simulink model "bipedal_robot"  (R2020b)
settings: Solver=ode23  StartTime=0.0  StopTime=TG.Tsim  MaxStep=0.01  RelTol=1e-3  AbsTol=1e-3  EnableMultiTasking=on
values from neighbouring files (symbols this model uses):
  cdf_data = zmp_cdf(foot,total_mass,0)    [bipedal.m]
  g = 9.80665    [bipedal.m]
  Tfil = Ts*10    (= 0.01)    [bipedal.m]
  total_mass = mlist(1) + ll_mass + rl_mass    [bipedal.m]
  Ts = 1/fs    (= 0.001)    [bipedal.m]
  use_reference_FBdata = 0    [bipedal.m]
undefined symbols (not defined in the file or in its folder): Base, ctrl_cfg_rem, ctrl_config, ctrl_data, foot, LefAnklePitch, LefAnkleRoll, LefHipPitch, LefHipRoll, LefHipYaw, LefKnee, lleg_FS_str, lleg_str, RigAnklePitch, RigAnkleRoll, RigHipPitch, RigHipRoll, RigHipYaw, RigKnee, rleg_FS_str, rleg_str, sim_floor, TG_test_type, X, Y, Z
libraries: sm_lib x49, biped_lib x36, nesl_utility x9, robotmaniplib x5, controller_lib x1, simulink x1, Contact_Forces_Lib x1
(part 3 of 3)

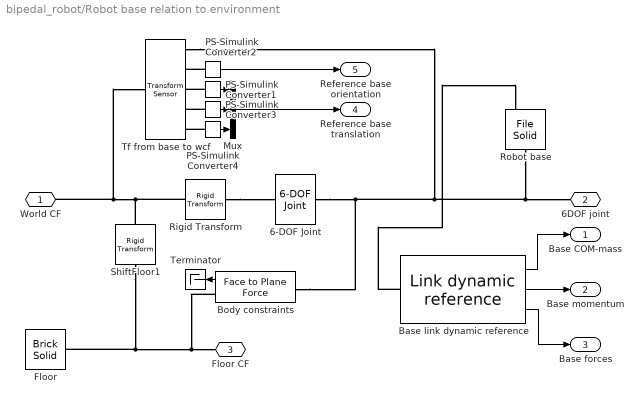
== system bipedal_robot/Robot base relation to environment ==
  6-DOF Joint : sm_lib/Joints/6-DOF Joint  JointMode=Normal  SenseConstraintForce=off  SenseConstraintForceX=off  SenseConstraintForceY=off  SenseConstraintForceZ=off  SenseConstraintTorque=off  SenseConstraintTorqueX=off  SenseConstraintTorqueY=off  SenseConstraintTorqueZ=off  SenseTotalForce=off  SenseTotalForceX=off  SenseTotalForceY=off  SenseTotalForceZ=off  SenseTotalTorque=off  SenseTotalTorqueX=off  SenseTotalTorqueY=off  SenseTotalTorqueZ=off  CompositeWrenchDir=FollowerOnBase  CompositeWrenchFrame=BaseFrame  PxEquilibriumPosition=0  PxEquilibriumPositionUnits=m  PxSpringStiffness=0  PxSpringStiffnessUnits=N/m  PxDampingCoefficient=0  PxDampingCoefficientUnits=N/(m/s)  PxTorqueActuationMode=NoTorque  PxMotionActuationMode=ComputedMotion  PxSensePosition=off  PxSenseVelocity=off  PxSenseAcceleration=off  PxSenseTorqueForce=off  PxSenseLowerLimitTorqueForce=off  PxSenseUpperLimitTorqueForce=off  PxLowerLimitSpecify=off  PxLowerLimitBound=-1  PxLowerLimitBoundUnits=m  PxLowerLimitStiffness=1e6  PxLowerLimitStiffnessUnits=N/m  PxLowerLimitDamping=1e3  PxLowerLimitDampingUnits=N/(m/s)  PxLowerLimitTransitionRegionWidth=1e-4  PxLowerLimitTransitionRegionWidthUnits=m  PxUpperLimitSpecify=off  PxUpperLimitBound=1  PxUpperLimitBoundUnits=m  PxUpperLimitStiffness=1e6  PxUpperLimitStiffnessUnits=N/m  PxUpperLimitDamping=1e3  PxUpperLimitDampingUnits=N/(m/s)  PxUpperLimitTransitionRegionWidth=1e-4  PxUpperLimitTransitionRegionWidthUnits=m  PxPositionTargetSpecify=on  PxPositionTargetPriority=High  PxPositionTargetValue=Base.Xinit(1)  PxPositionTargetValueUnits=m  PxVelocityTargetSpecify=off  PxVelocityTargetPriority=High  PxVelocityTargetValue=0  PxVelocityTargetValueUnits=m/s  PyEquilibriumPosition=0  PyEquilibriumPositionUnits=m  PySpringStiffness=0  PySpringStiffnessUnits=N/m  PyDampingCoefficient=0  PyDampingCoefficientUnits=N/(m/s)  PyTorqueActuationMode=NoTorque  PyMotionActuationMode=ComputedMotion  PySensePosition=off  PySenseVelocity=off  PySenseAcceleration=off  PySenseTorqueForce=off  PySenseLowerLimitTorqueForce=off  PySenseUpperLimitTorqueForce=off  PyLowerLimitSpecify=off  PyLowerLimitBound=-1  PyLowerLimitBoundUnits=m  PyLowerLimitStiffness=1e6  PyLowerLimitStiffnessUnits=N/m  PyLowerLimitDamping=1e3  PyLowerLimitDampingUnits=N/(m/s)  PyLowerLimitTransitionRegionWidth=1e-4  PyLowerLimitTransitionRegionWidthUnits=m  PyUpperLimitSpecify=off  PyUpperLimitBound=1  PyUpperLimitBoundUnits=m  PyUpperLimitStiffness=1e6  PyUpperLimitStiffnessUnits=N/m  PyUpperLimitDamping=1e3  PyUpperLimitDampingUnits=N/(m/s)  PyUpperLimitTransitionRegionWidth=1e-4  PyUpperLimitTransitionRegionWidthUnits=m  PyPositionTargetSpecify=on  PyPositionTargetPriority=High  PyPositionTargetValue=Base.Xinit(2)  PyPositionTargetValueUnits=m  PyVelocityTargetSpecify=off  PyVelocityTargetPriority=High  PyVelocityTargetValue=0  PyVelocityTargetValueUnits=m/s  PzEquilibriumPosition=0  PzEquilibriumPositionUnits=m  PzSpringStiffness=0  PzSpringStiffnessUnits=N/m  PzDampingCoefficient=0  PzDampingCoefficientUnits=N/(m/s)  PzTorqueActuationMode=NoTorque  PzMotionActuationMode=ComputedMotion  PzSensePosition=off  PzSenseVelocity=off  PzSenseAcceleration=off  PzSenseTorqueForce=off  PzSenseLowerLimitTorqueForce=off  PzSenseUpperLimitTorqueForce=off  PzLowerLimitSpecify=off  PzLowerLimitBound=0  PzLowerLimitBoundUnits=m  PzLowerLimitStiffness=1e6  PzLowerLimitStiffnessUnits=N/m  PzLowerLimitDamping=1e3  PzLowerLimitDampingUnits=N/(m/s)  PzLowerLimitTransitionRegionWidth=1e-4  PzLowerLimitTransitionRegionWidthUnits=m  PzUpperLimitSpecify=off  PzUpperLimitBound=1  PzUpperLimitBoundUnits=m  PzUpperLimitStiffness=1e6  PzUpperLimitStiffnessUnits=N/m  PzUpperLimitDamping=1e3  PzUpperLimitDampingUnits=N/(m/s)  PzUpperLimitTransitionRegionWidth=1e-4  PzUpperLimitTransitionRegionWidthUnits=m  PzPositionTargetSpecify=on  PzPositionTargetPriority=High  PzPositionTargetValue=Base.Xinit(3)  PzPositionTargetValueUnits=m  PzVelocityTargetSpecify=off  PzVelocityTargetPriority=High  PzVelocityTargetValue=0  PzVelocityTargetValueUnits=m/s  SphDefPosRotationMethod=None  SphDefPosRotationAngleUnits=deg  SphDefPosRotationStandardAxis=+Z  SphDefPosRotationAngle=0.0  SphDefPosRotationArbitraryAxis=[0 0 1]  SphDefPosFollAlignAxisA=+X  SphDefPosBaseAlignAxisA=+Y  SphDefPosFollAlignAxisB=+Y  SphDefPosBaseAlignAxisB=+Z  SphDefPosRotationSequenceAxes=FollowerAxes  SphDefPosRotationSequence=XYX  SphDefPosRotationSequenceAngles=[0 0 0]  SphDefPosRotationSequenceAnglesUnits=deg  SphDefPosRotationMatrix=[1 0 0; 0 1 0; 0 0 1]  SphEqPosRotationMethod=None  SphEqPosRotationAngleUnits=deg  SphEqPosRotationStandardAxis=+Z  SphEqPosRotationAngle=0.0  SphEqPosRotationArbitraryAxis=[0 0 1]  SphEqPosFollAlignAxisA=+X  SphEqPosBaseAlignAxisA=+Y  SphEqPosFollAlignAxisB=+Y  SphEqPosBaseAlignAxisB=+Z  SphEqPosRotationSequenceAxes=FollowerAxes  SphEqPosRotationSequence=XYX  SphEqPosRotationSequenceAngles=[0 0 0]  SphEqPosRotationSequenceAnglesUnits=deg  SphEqPosRotationMatrix=[1 0 0; 0 1 0; 0 0 1]  SphSpringStiffness=0  SphSpringStiffnessUnits=N*m/deg  SphDampingCoefficient=0  SphDampingCoefficientUnits=N*m/(deg/s)  SphActuateTorqueX=off  SphActuateTorqueY=off  SphActuateTorqueZ=off  SphActuateTorque=off  SphTorqueActuationMode=NoTorque  SphMotionActuationMode=ComputedMotion  SphActuationFrame=BaseFrame  SphSensePosition=off  SphSenseVelocityX=off  SphSenseVelocityY=off  SphSenseVelocityZ=off  SphSenseVelocity=off  SphSenseAccelerationX=off  SphSenseAccelerationY=off  SphSenseAccelerationZ=off  SphSenseAcceleration=off  SphSenseTorqueX=off  SphSenseTorqueY=off  SphSenseTorqueZ=off  SphSenseTorqueForce=off  SphSenseLowerLimitTorqueMag=off  SphSenseUpperLimitTorqueMag=off  SphSensingFrame=BaseFrame  SphLowerLimitSpecify=off  SphLowerLimitBound=15  SphLowerLimitBoundUnits=deg  SphLowerLimitStiffness=1e4  SphLowerLimitStiffnessUnits=N*m/deg  SphLowerLimitDamping=10  SphLowerLimitDampingUnits=N*m/(deg/s)  SphLowerLimitTransitionRegionWidth=0.1  SphLowerLimitTransitionRegionWidthUnits=deg  SphUpperLimitSpecify=off  SphUpperLimitBound=45  SphUpperLimitBoundUnits=deg  SphUpperLimitStiffness=1e4  SphUpperLimitStiffnessUnits=N*m/deg  SphUpperLimitDamping=10  SphUpperLimitDampingUnits=N*m/(deg/s)  SphUpperLimitTransitionRegionWidth=0.1  SphUpperLimitTransitionRegionWidthUnits=deg  SphPositionTargetRotationMethod=StandardAxis  SphPositionTargetRotationAngleUnits=rad  SphPositionTargetRotationStandardAxis=+Y  SphPositionTargetRotationAngle=0  SphPositionTargetRotationArbitraryAxis=[0 0 1]  SphPositionTargetFollAlignAxisA=+X  SphPositionTargetBaseAlignAxisA=+Y  SphPositionTargetFollAlignAxisB=+Y  SphPositionTargetBaseAlignAxisB=+Z  SphPositionTargetRotationSequenceAxes=FollowerAxes  SphPositionTargetRotationSequence=XYX  SphPositionTargetRotationSequenceAngles=[0 0 0]  SphPositionTargetRotationSequenceAnglesUnits=deg  SphPositionTargetRotationMatrix=[1 0 0; 0 1 0; 0 0 1]  SphPositionTargetSpecify=on  SphPositionTargetPriority=High  SphVelocityTargetValue=[0 0 0]  SphVelocityTargetValueUnits=deg/s  SphVelocityTargetSpecify=off  SphVelocityTargetPriority=High  SphVelocityTargetInFollowerFrame=on
  Base link dynamic reference : biped_lib/Link dynamic reference  M=Base.body.mass  I=Base.body.inertia
  Body constraints : Contact_Forces_Lib/3D/Composite Forces/Face to Plane Force  PlaB_x=sim_floor.dims(1)  PlaB_y=sim_floor.dims(2)  PlaB_z=sim_floor.dims(3)/2  FacF_x=Base.dims(1)  FacF_y=Base.dims(2)  FacF_z=Base.dims(3)/2  FacF_rSph=0.01  force_law_pla2pla=Linear  k_contact_pla2pla=Kcont  b_contact_pla2pla=Dcont  pen_full_damp_F_pla2pla=1e-4  pen_exponent_pla2pla=1  friction_law_pla2pla=Stick-Slip Continuous  mu_kinetic_pla2pla=0.5  mu_static_pla2pla=0.7  v_thr_pla2pla=0.001  vis_on_pla2pla=off  vis_opc_en_box2box=0  vis_len_plaLz=0.005  vis_clr=[0.9 0.2 0.2]  vis_opc=0.7
      settings: SourceProductName=Simscape Multibody Contact Forces Library
  Floor : sm_lib/Body Elements/Brick Solid  GraphicAmbientColor=[0.15 0.15 0.15 1.0]  BasedOnType=Density  BrickDimensions=sim_floor.dims  BrickDimensionUnits=m  CenterOfMass=[0 0 0]  CenterOfMassUnits=m  GraphicDiffuseColor=[0.8 0.8 0.8]  Density=1000  DensityUnits=kg/m^3  DoExposeReferenceFrame=on  GraphicEmissiveColor=[0.0 0.0 0.0 1.0]  ExportEntireGeometry=off  SerializedFrames=<Frames/>  MarkerShape=Sphere  MarkerSize=10  GraphicType=FromGeometry  InertiaType=CalculateFromGeometry  Mass=1  MassUnits=kg  MomentsOfInertia=[1 1 1]  MomentsOfInertiaUnits=kg*m^2  GraphicOpacity=1.0  ProductsOfInertia=[0 0 0]  ProductsOfInertiaUnits=kg*m^2  GraphicShininess=75  GraphicSpecularColor=[0.5 0.5 0.5 1.0]  GraphicVisPropType=SimpleVisualProperties
      settings: SourceProductName=Multibody
  Mux : Mux  Inputs=3
  PS-Simulink Converter{1..4} (4 alike) : nesl_utility/PS-Simulink Converter  PhysicalDomain=network_engine_domain  SubClassName=ps_output  LeftPortType=input  RightPortType=output  PseudoPeriodic=off  Frequencies=[]  Unit=1  AffineConversion=off
  Rigid Transform : sm_lib/Frames and Transforms/Rigid Transform  TranslationMethod=StandardAxis  TranslationStandardOffset=0  TranslationLengthUnit=m  TranslationStandardAxis=+Z  TranslationCartesianOffset=[0 0 0]  TranslationROffset=0  TranslationROffsetUnits=m  TranslationZOffset=0  TranslationZOffsetUnits=m  TranslationThetaOffset=0  TranslationThetaOffsetUnits=deg  RotationMethod=None  RotationAngleUnits=deg  RotationStandardAxis=+Z  RotationAngle=0.0  RotationArbitraryAxis=[0 0 1]  FollAlignAxisA=+X  BaseAlignAxisA=+Y  FollAlignAxisB=+Y  BaseAlignAxisB=+Z  RotationSequenceAxes=FollowerAxes  RotationSequence=XYX  RotationSequenceAngles=[0 0 0]  RotationSequenceAnglesUnits=deg  RotationMatrix=[1 0 0; 0 1 0; 0 0 1]
  Robot base : sm_lib/Body Elements/File Solid  ExtGeomFileName=Base.stl  UnitType=Custom  ExtGeomFileUnits=mm  StepReaderType=HEX  ExportConvexHullGeometry=on  InertiaType=Custom  Mass=Base.body.mass  MassUnits=kg  CenterOfMass=Base.body.com  CenterOfMassUnits=m  MomentsOfInertia=Base.body.inertia(1:3)  MomentsOfInertiaUnits=kg*m^2  ProductsOfInertia=Base.body.inertia(4:6)  ProductsOfInertiaUnits=kg*m^2  BasedOnType=Mass  Density=1000  DensityUnits=kg/m^3  DoExposeReferenceFrame=on  SerializedFrames=<Frames><Frame><Id>Frame1</Id><Value><Name>COM</Name><Origin><Source>CenterOfMassFrame</Source><FeatureName></FeatureName></Origin><PrimaryAxis><DefinedDirection>+Z</DefinedDirection><Source>ReferenceFrame</Source><SourceDirection>+Z</SourceDirection><FeatureName></FeatureName></PrimaryAxis><SecondaryAxis><DefinedDirection>+X</DefinedDirection><Source>ReferenceFrame</Source><SourceDirection>+X</SourceDirection><FeatureName></FeatureName></SecondaryAxis></Value></Frame></Frames>  GraphicType=FromGeometry  MarkerShape=Sphere  MarkerSize=10  GraphicVisPropType=SimpleVisualProperties  GraphicDiffuseColor=[0.5 0.5 0.5]  GraphicSpecularColor=[0.5 0.5 0.5 1.0]  GraphicAmbientColor=[0.15 0.15 0.15 1.0]  GraphicEmissiveColor=[0.0 0.0 0.0 1.0]  GraphicShininess=75  GraphicOpacity=1.0
  ShiftFloor1 : sm_lib/Frames and Transforms/Rigid Transform  TranslationMethod=StandardAxis  TranslationStandardOffset=-sim_floor.dims(3)/2  TranslationLengthUnit=m  TranslationStandardAxis=+Z  TranslationCartesianOffset=[0 0 0]  TranslationROffset=0  TranslationROffsetUnits=m  TranslationZOffset=0  TranslationZOffsetUnits=m  TranslationThetaOffset=0  TranslationThetaOffsetUnits=deg  RotationMethod=None  RotationAngleUnits=deg  RotationStandardAxis=+Z  RotationAngle=0.0  RotationArbitraryAxis=[0 0 1]  FollAlignAxisA=+X  BaseAlignAxisA=+Y  FollAlignAxisB=+Y  BaseAlignAxisB=+Z  RotationSequenceAxes=FollowerAxes  RotationSequence=XYX  RotationSequenceAngles=[0 0 0]  RotationSequenceAnglesUnits=deg  RotationMatrix=[1 0 0; 0 1 0; 0 0 1]
  Terminator : Terminator
  Tf from base to wcf : sm_lib/Frames and Transforms/Transform Sensor  MeasurementFrame=World  SenseAngle=off  SenseAxis=off  SenseAngle1=off  SenseAngle2=off  SenseAngle3=off  SenseQ=off  SenseR=on  SenseOmegaX=off  SenseOmegaY=off  SenseOmegaZ=off  SenseOmega1=off  SenseOmega2=off  SenseOmega3=off  SenseQDot=off  SenseRDot=off  SenseAlphaX=off  SenseAlphaY=off  SenseAlphaZ=off  SenseAlpha1=off  SenseAlpha2=off  SenseAlpha3=off  SenseQDDot=off  SenseRDDot=off  SenseX=on  SenseY=on  SenseZ=on  SenseRad=off  SenseAzim=off  SenseDist=off  SenseInc=off  SenseXDot=off  SenseYDot=off  SenseZDot=off  SenseRadDot=off  SenseAzimDot=off  SenseDistDot=off  SenseIncDot=off  SenseXDDot=off  SenseYDDot=off  SenseZDDot=off  SenseRadDDot=off  SenseAzimDDot=off  SenseDistDDot=off  SenseIncDDot=off
  World CF : PMIOPort  Side=Left
  6DOF joint : PMIOPort  Port=2  Side=Right
  Floor CF : PMIOPort  Port=3  Side=Right
  Base COM-mass : Outport
  Base momentum : Outport  Port=2
  Base forces : Outport  Port=3
  Reference base translation : Outport  Port=4
  Reference base orientation : Outport  Port=5
  wires:
  Body constraints/1 -> Terminator/1
  Base link dynamic reference/1 -> Base COM-mass/1
  Base link dynamic reference/2 -> Base momentum/1
  Base link dynamic reference/3 -> Base forces/1
  PS-Simulink Converter2/1 -> Reference base orientation/1
  PS-Simulink Converter3/1 -> Mux/2
  PS-Simulink Converter1/1 -> Mux/1
  PS-Simulink Converter4/1 -> Mux/3
  Mux/1 -> Reference base translation/1
  connections:
  Rigid Transform/LConn1 -- Tf from base to wcf/LConn1 -- World CF/RConn1 -- ShiftFloor1/LConn1
  Rigid Transform/RConn1 -- 6-DOF Joint/LConn1
  6-DOF Joint/RConn1 -- Body constraints/LConn1 -- Tf from base to wcf/RConn1 -- Robot base/RConn1 -- 6DOF joint/RConn1
  ShiftFloor1/RConn1 -- Floor/RConn1 -- Floor CF/RConn1 -- Body constraints/RConn1
  PS-Simulink Converter2/LConn1 -- Tf from base to wcf/RConn2
  PS-Simulink Converter1/LConn1 -- Tf from base to wcf/RConn3
  PS-Simulink Converter3/LConn1 -- Tf from base to wcf/RConn4
  PS-Simulink Converter4/LConn1 -- Tf from base to wcf/RConn5
  Base link dynamic reference/LConn1 -- Robot base/LConn1

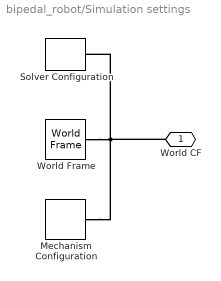
== system bipedal_robot/Simulation settings ==
  Mechanism Configuration : sm_lib/Utilities/Mechanism Configuration  UniformGravity=Constant  GravityVector=gvec  GravityVectorUnits=m/s^2  GravityUnits=m/s^2  LinearizationDelta=0.001  JointModeTransitionNonlinearIterations=2
      settings: SourceProductName=Multibody
  Solver Configuration : nesl_utility/Solver Configuration  PhysicalDomain=network_engine_domain  SubClassName=solver  LeftPortType=input  RightPortType=generic  Tones=[]  Harmonics=[]  SimulateNoise=off  Profile=off  UseLocalSampling=off  EnableSwitchedLinearOptims=on  FrequencyDomain=off  UseCCode=off  RelTol=0.001  AbsTol=1e-06  MinStep=1e-09  ToWorkspace=off  RevertToSquareIcSolve=off  NumHomotopyIterations=100  PhasorMode=off  PhasorModeNumHarmonics=1  DoDC=off  ResidualTolerance=1e-09  UseLocalSolver=off  LocalSolverChoice=NE_BACKWARD_EULER_ADVANCER  LocalSolverSampleTime=0.001  DoFixedCost=off  MaxNonlinIter=3  MaxModeIter=2  ComputeImpulses=off  ImpulseIterations=2  LinearAlgebra=Sparse  EquationFormulation=NE_TIME_EF  DelaysMemoryBudget=1024  AutomaticFiltering=on  FilteringTimeConstant=0.001  PartitionStorageMethod=AS_NEEDED  PartitionMemoryBudget=1024  PartitionMethod=FAST
      settings: SourceProductName=Utilities
  World Frame : sm_lib/Frames and Transforms/World Frame
      settings: SourceProductName=Multibody
  World CF : PMIOPort  Side=Right
  connections:
  World Frame/RConn1 -- World CF/RConn1 -- Solver Configuration/RConn1 -- Mechanism Configuration/RConn1

== matlab function bipedal_robot/Controller/Sensor mapping ==
  data: MSL input; Qconfig output; MSR input
function Qconfig = fcn(MSL,MSR)
    [LL,RL] = group_motor_data(MSL,MSR);
    Qconfig = zeros(12,1);
    %joints start at hip and go down to ankle. Left and right joints are
    %always following one another
    Qconfig(1:2:end) = LL.q;
    Qconfig(2:2:end) = RL.q;
    %if using roby
    %Qconfig(1:end/2) = LL.q;
    %Qconfig(end/2+1:end) = RL.q;

== matlab function bipedal_robot/Controller/Walking controller ==
  data: time input; MSL input; TL output; FSL input; MSR input; FSR input; ZMP_ref input; TR output; COM_des output; p_des output; COM_ref input; ctrl_data input; ctrl_config input; twb input; Rwb input; GenMotion input; p_ref output; p_qp output; dcm_des output; dcm_meas output; test_type input; e_qL output; e_qR output; zL_glo output; zR_glo output; COMDat output; p_meas output
function [TL,TR, COM_des, p_des, p_ref, p_qp, dcm_des, dcm_meas, e_qL, e_qR, zL_glo, zR_glo,COMDat,p_meas] = fcn(time, MSL, FSL, MSR, FSR, ZMP_ref, COM_ref, ctrl_data, ctrl_config, twb, Rwb, GenMotion, test_type)
persistent dcm_int;
persistent init_corr corr_stored cz_int;
persistent C_obs_old Cp_obs_old;

%% constants & configuration
dt = 1/ctrl_config.fctrl;
z_des = ctrl_config.com_height;
g = 9.81;
omega = sqrt(g/z_des);
zp_des = 0;
Mtot = ctrl_config.mass;
mlist = ctrl_config.mlist;
foot_data = ctrl_config.foot_data;
foot_dims = foot_data.dims(1:2)*0.9;
K = Mtot*omega^2;
damper_model = ctrl_config.damper;

%% memory variables
if isempty(dcm_int)
    cz_int = 0;
    dcm_int = zeros(2,1); %initialise the integrator
    corr_stored = zeros(3,1);
    C_obs_old = [GenMotion(6:7);z_des]; %prevents controller jumps
    Cp_obs_old = zeros(3,1);
end



%% values from the pattern generator
if test_type == 0
    %only stabilization (trajectories are not used) => disturbance test
    phase = 0; %DS all the time
    WshiftL = 0.5; %equal wrench distribution
    WshiftR = 0.5;
    ZMP_des = ctrl_config.pdes_ini;
    COM_des = ZMP_des;
    COMp_des = zeros(2,1);
    qL_des = ctrl_config.qLd;
    qR_des = ctrl_config.qRd;
    qLp_des = zeros(6,1);
    qRp_des = zeros(6,1);
else
    % all the other tests require a trajectory
    if test_type == 1
        % shifting the weight only
        phase = 0;  % always remain in DS phase
    else
        % lifting the swing leg
        phase = GenMotion(1);
    end
    WshiftL = GenMotion(2);
    WshiftR = GenMotion(3);
    ZMP_des = GenMotion(4:5);
    COM_des = GenMotion(6:7);
    COMp_des = GenMotion(8:9);
    qL_des = GenMotion(10:15);
    qR_des = GenMotion(16:21);
    qLp_des = GenMotion(22:27);
    qRp_des = GenMotion(28:33);
end

%% Desired state values
activate_foot_adaptation = 0;
[qLdes_new,qRdes_new,qLp_des_new,qRp_des_new] = foot_tilt_ctrl(FSL.Fm, FSR.Fm, qL_des, qR_des, qLp_des, qRp_des, dt, activate_foot_adaptation);

%desired joint angles
qLd = qLdes_new;%qLd = ctrl_config.qLd;
qRd = qRdes_new;%qRd = ctrl_config.qRd;
%desired joint velocities
qLpd = qLp_des_new;
qRpd = qRp_des_new;
% desired ZMP
p_des = ZMP_des; %p_des = ctrl_config.pdes_ini(1:2) + dcm_offs;
% desired COM
C_d = COM_des;%C_d = p_des;zeros(3,1);
Cp_d = COMp_des;%Cp_d = [0,0]';
% desired DCM
dcm_des = C_d + Cp_d/omega;


%% Measurements from motors
[LL,RL] = group_motor_data(MSL,MSR);
qL = LL.q;
qR = RL.q;
qLp = LL.qp;
qRp = RL.qp;

%% COM & ZMP observer (Now: FB estimation implemented - missing: COM velocity estimation)
% ZMP observer
Hwb = [
    Rwb,twb;
    zeros(1,3),1;
];

Hw_eeL = Hwb / ctrl_data.TL;
Hw_eeR = Hwb / ctrl_data.TR;
[zmp_glo_Comp,zL_Comp,zR_Comp] = compute_zmp_full(FSL, FSR, foot_data, Hw_eeL, Hw_eeR, 1, 0); %computed zmp
zL_glo = zL_Comp.glo;
zR_glo = zR_Comp.glo;

% COM observer
fb_tra_Comp = twb;
fb_rot_Comp = rotm2eul(Rwb,"xyz")';
xfb = [fb_tra_Comp;fb_rot_Comp];
C_obs = compute_com_pos2(xfb,qL,qR,mlist,'w');
% low pass filter the velocity
alphaCOM = 0.05;
Cp_obs = alphaCOM * (C_obs - C_obs_old)/dt + (1 - alphaCOM) * Cp_obs_old;
%overwrite old values
C_obs_old = C_obs;
Cp_obs_old = Cp_obs;


%Reference values
if time<0.2
    C_meas = COM_ref(1:3);
    Cp_meas = COM_ref(4:6);
else
    C_meas = C_obs;
    Cp_meas = Cp_obs;
end

COMDat = [COM_ref(1:3);C_obs;COM_ref(4:6);Cp_obs];

use_zmp_ref = 0;
if use_zmp_ref
    p_meas = ZMP_ref;
else
    p_meas = zmp_glo_Comp; %works reliably now (the problem was a wrong Tf)
end


%%%%%%% THIS PART HAS TO BE ADAPTED NEXT WEEK. DEPENDING ON THE SELECTED
%%%%%%% OPTION, EITHER TORQUE CONTROL OR POSITION CONTROL IS CHOSEN. FOR
%%%%%%% POSITION CONTROL THERE SHOULD BE ONE OPTION TO USE ADMITTANCE
%%%%%%% TO MAP THE TORQUE CONTROL INTO ACCELERATION AND THEN INTEGRATE IT
%%%%%%% TO GET VELOCITY TARGETS NEEDED BY THE OPTIMIZATION.

%% COM controller 
% gain setup
sc = omega;
Kp_com = [1.6*sc;1.3*sc];
Kp_comz = 1000*sc;
Kd_comz = 400*sc;
Ki_comz = 3000*sc;
Kp_p = [0.2*sc;0.2*sc];

% leaky integrator
Ki_com = [1*sc;1*sc];
Kleak = [0.1;0.1];

% control law for COM forces
if C_meas(3)==0
    czerr = 0;
    C_meas_ada = C_meas;
else
    if isempty(init_corr)
        init_corr = 1;
        %corr_stored = C_meas - [0;0;z_des];
    end
    C_meas_ada = C_meas - [0,0,corr_stored(3)]'; %this will have to be performed in practice as well
    
    cz_err = z_des-C_meas_ada(3);
    cz_int = cz_int + dt*cz_err;
    
    czerr = Kd_comz*(zp_des - Cp_meas(3)) + Kp_comz*cz_err + Ki_comz*cz_int;
end

%% DCM observer
dcm_meas = C_meas_ada(1:2) + C_meas_ada(1:2)/omega;
% integrate the DCM error (IIR filter)
dT = 1/ctrl_config.fctrl;
dcm_err = dcm_des - dcm_meas; %integral error
d_err = dcm_err - Kleak.*dcm_int; %inclusion of leakage
dcm_int = dcm_int + dT * d_err;

%% CONTROLLER
% reference value for the ZMP
p_ref = p_des -(1+Kp_com./omega).*dcm_err - Ki_com./omega.*dcm_int + Kp_p./omega.*(p_des-p_meas);

% force
Fd = [
    -K*(C_meas_ada(1)-p_ref(1));
    -K*(C_meas_ada(2)-p_ref(2));
    -(Mtot*g + czerr);
];

% control law for torques around COM
% angular velocities measured in motors attached rigidly to base (M1 - L&R)
%left measurement
w_1L = LL.w(:,1);
R_base_IMU_1L = rotz(-pi/6);
wbaseL = R_base_IMU_1L*w_1L;
%right measurement
w_1R = RL.w(:,1);
R_base_IMU_1R = rotz(+pi/6);
wbaseR = R_base_IMU_1R*w_1R;
%average both
omega=(wbaseL+wbaseR)/2;
omega_w = Rwb*omega; %express the locally measured rot. velocity in the world frame
Td = floating_base_orientation(Rwb',omega_w); %transpose the rotm to get the correct mapping (FROM:desired TO:actual)
%Td = zeros(3,1);
% generate an overall wrench (in the world frame)
Wc = [Fd;Td]; 

% get jaccobians 
% WATCH OUT => First lines 1-3 are Jw and 4-6 are Jv (swapped rot. and tr.
% motion)
JL = ctrl_data.JL(:,1:2:end); 
JLcorr = [JL(4:6,:);JL(1:3,:)];

JR = ctrl_data.JR(:,2:2:end);
JRcorr = [JR(4:6,:);JR(1:3,:)];

% get transformations (feet to base)
TF_world_base = [
    Rwb, twb;
    zeros(1,3),1
];

TF_world_com = [
    eye(3),C_meas;
    zeros(1,3),1
];

TF_com_base = TF_world_com\TF_world_base; %TF from base to COM

TF_base_eeL = ctrl_data.TL; %TF from left end effector to base
TF_base_eeR = ctrl_data.TR; %TF from right end effector to base

% get required wrench mappings
AdT_gcb = Ad_g(TF_com_base(1:3,1:3),TF_com_base(1:3,4))';
AdT_gbl = Ad_g(TF_base_eeL(1:3,1:3),TF_base_eeL(1:3,4))';
AdT_gbr = Ad_g(TF_base_eeR(1:3,1:3),TF_base_eeR(1:3,4))';

%% torque distribution
% transform the wrench from com to the body frame (gcb transforms vectors
% from base to com, but AdT is dual - transforms in the oposite order)
%Wb = AdT_gcb*Wc;
% equally distribute the wrench and transform them to the feet frames
%Wlfoot = AdT_gbl*Wb /2;
%Wrfoot = AdT_gbr*Wb /2;
[Wlfoot,Wrfoot] = distribute_wrench_tracking(Wc,JLcorr,JRcorr,TF_com_base,TF_base_eeL,TF_base_eeR,foot_dims,0.6,0,phase,WshiftL,WshiftR);
% map the wrenches to respective joint torques
TLtc = JLcorr'*Wlfoot;
TRtc = JRcorr'*Wrfoot;


%% Test if the zmp recomputation matters
TF_world_eeL = TF_world_base*inv(TF_base_eeL);
TF_world_eeR = TF_world_base*inv(TF_base_eeR);
RwL = TF_world_eeL(1:3,1:3);
RwR = TF_world_eeR(1:3,1:3);
twL = TF_world_eeL(1:3,4);
twR = TF_world_eeR(1:3,4);
[pL,Wlfoot_rot] = zmp_from_wrench(Wlfoot,RwL,twL);
[pR,Wrfoot_rot] = zmp_from_wrench(Wrfoot,RwR,twR);
p_qp = (Wlfoot_rot(3)*pL+Wrfoot_rot(3)*pR)/(Wlfoot_rot(3)+Wrfoot_rot(3));

%% Joint control (secondary task)
[KpL, KpR, KdL, KdR] = get_gains(test_type, phase, WshiftL, WshiftR);

% compute errors
e_qL = qLd-qL;
e_qR = qRd-qR;
ep_qL = qLpd-qLp;
ep_qR = qRpd-qRp;
% separated pd control
TLpos = KpL.*e_qL;
TRpos = KpR.*e_qR;
TLvel = KdL.*ep_qL;
TRvel = KdR.*ep_qR;

% Null space projector (for a 2 level hierarchy, successive and augmented projectors are the same)
use_NS_ctrl = 2;
if use_NS_ctrl && phase == 0 %can only be used in DS phase
    rho = 0.1; %needs to be included
    Jfull = [JLcorr,JRcorr];
    JLpseud = pseudoinv(Jfull,rho,'right');
    % compute the projector
    Nproj2 = (eye(12)-Jfull'*JLpseud');
    % project the secondary task to the nullspace of the primary one
    if use_NS_ctrl==1
        %only position is projected 
        Tsec = Nproj2*[TLpos;TRpos];
        TLsec = Tsec(1:end/2);
        TRsec = Tsec(end/2+1:end);
        %velocity is added
        TLsec = TLsec + TLvel;
        TRsec = TRsec + TLvel;
    elseif use_NS_ctrl==2
        %position and velocity are projected
        Tsec = Nproj2*[TLpos+TLvel;TRpos+TRvel];
        TLsec = Tsec(1:end/2);
        TRsec = Tsec(end/2+1:end);
    end
else
    % simply add the secondary task to the primary on
    TLsec = TLpos + TLvel;
    TRsec = TRpos + TLvel;
    if phase == 1
        Grem = rtbox_to_alg(ctrl_data.G);
        Gl = Grem(1:end/2);
        Gr = Grem(end/2+1:end);
        if WshiftL>WshiftR
            %right leg is swinging
            TRsec = TRsec + Gr;
        else
            %left leg is swinging
            TLsec = TLsec + Gl;
        end
    end
end


[TLdamp, TRdamp] = damperCompensTorques(qL,qR,damper_model);
    

%% Combined control
TL = TLtc + TLsec + TLdamp;
TR = TRtc + TRsec + TRdamp;

== matlab function bipedal_robot/Controller/Fl. base est. ==
  data: pest_w_b output; Rest_w_b output; time input; Hest_w_b output; MSL input; LFL input; MSR input; LFR input; GenMotion input; cdf_data input; FS_ref input; FootDataPmeas input
function [pest_w_b,Rest_w_b,Hest_w_b]  = fcn(time, MSL, LFL, MSR, LFR, GenMotion, cdf_data, FS_ref, FootDataPmeas)
persistent init Hw_L_corr Hw_R_corr;
persistent quatLimu_old quatRimu_old;
persistent quatLimu_old2 quatRimu_old2;

%joint angles from the trajectory generator
qL_tg = GenMotion(10:15);
qR_tg = GenMotion(16:21);
%leg to base transformations from tg
[HLlist_tg] = H_abs_bL(qL_tg);
[HRlist_tg] = H_abs_bR(qR_tg);
%tf from ee to base from tg
Hb_eeL_tg = reshape(HLlist_tg(end,:,:),4,4);
Hb_eeR_tg = reshape(HRlist_tg(end,:,:),4,4);
%feet positions in the world frame
pw_eeL = GenMotion(34:36);
pw_eeR = GenMotion(37:39);

%since in the ideal case, base frame coincides with the world
%frame  when it comes to orientation, ee->base is taken as known rotation
%between ee->world (IF BASE TRAJECTORY WOULD HAVE VARYING ORIENTATION, THIS
%WOULD HAVE TO BE CORRECTED)
Hw_eeL = [
    Hb_eeL_tg(1:3,1:3),pw_eeL;
    zeros(1,3),1;
];

Hw_eeR = [
    Hb_eeR_tg(1:3,1:3),pw_eeR;
    zeros(1,3),1;
];

%begin by not doing any compensation (IMU has no bias yet)
compensate_drift = 0; 
if isempty(init)
    init = 1;
    %only executed at the init phase
    Hw_L_corr = Hw_eeL;
    Hw_R_corr = Hw_eeR;
    
    quatLimu_old = [1;0;0;0];
    quatRimu_old = quatLimu_old;
    quatLimu_old2 = quatLimu_old;
    quatRimu_old2 = quatLimu_old;
elseif compensate_drift
    %if the drift compensation is activated, this is executed every time
    Hw_eeL = Hw_L_corr;
    Hw_eeR = Hw_R_corr;
end

%% Measurements from motors
[LL,RL] = group_motor_data(MSL,MSR);
qL = LL.q;
qR = RL.q;
qLp = LL.qp;
qRp = RL.qp;
aL = LL.a;
aR = RL.a;
wL = LL.w;
wR = RL.w;

%% IMU based rotation estimation
%two imu-s that are rigidly attached to the floating base
R_b_imu1L = rotz(-pi/6);
R_b_imu1R = rotz(+pi/6);

%measurements from those two imus
a1Limu = aL(:,1);
a1Rimu = aR(:,1);
w1Limu = wL(:,1);
w1Rimu = wR(:,1);

%represent measurements in the base frame (just allignment, not spatial
%transformation - this means, that we are still working with the
%acceleration experienced at the position of the IMU)
a1Lb = R_b_imu1L*a1Limu;
a1Rb = R_b_imu1R*a1Rimu;
w1Lb = R_b_imu1R*w1Limu;
w1Rb = R_b_imu1R*w1Rimu;

%sampling rate
dt = 0.002;
%use the magdwick algorithm to obtain the estimated rotation in the wcf
%left
quatLimu = filter_update(a1Lb, w1Lb, quatLimu_old);
quatLimu_old = quatLimu;

quatLimu2 = rotm2quat(direct_fb_estimation(quat2rotm(quatLimu_old2'), a1Lb, w1Lb, dt))';
%overwrite old values
quatLimu_old2 = quatLimu2;

%right
quatRimu = filter_update(a1Rb, w1Rb, quatRimu_old);
quatRimu_old = quatRimu; 
    
quatRimu2 = rotm2quat(direct_fb_estimation(quat2rotm(quatRimu_old2'), a1Rb, w1Rb, dt))';
quatRimu_old2 = quatRimu2;

%measurements can not be merged directly, as they were obtained in
%different frames. Calculated quaternions however can be merged, as they
%are representing the rotation of the same body.
%averaging rotation matrices - Henze and Ott - documented in 3.2 FB pose
%est.
quat_imu_sum = (quatLimu+quatRimu)/2;
quat_imu_merged = quat_imu_sum/norm(quat_imu_sum); %orientation from the accelerometer
Rw_b_imu = quat2rotm(quat_imu_merged');

%% kinematics based rotation estimation
%fkine from the measured values
[HLlist] = H_abs_bL(qL);
[HRlist] = H_abs_bR(qR);
Hb_eeL = reshape(HLlist(end,:,:),4,4);
Hb_eeR = reshape(HRlist(end,:,:),4,4);
%translations which are needed for later
pb_eeL = Hb_eeL(1:3,4);
pb_eeR = Hb_eeR(1:3,4);

%kinematic guess for the transformation between wcf and base 
Hw_b_Lleg = Hw_eeL/Hb_eeL;
Hw_b_Rleg = Hw_eeR/Hb_eeR;

%rotations
Rw_b_Lleg = Hw_b_Lleg(1:3,1:3);
Rw_b_Rleg = Hw_b_Rleg(1:3,1:3);
%translations
pw_b_Lleg = Hw_b_Lleg(1:3,4);
pw_b_Rleg = Hw_b_Rleg(1:3,4);

%% fuse all three measurements depending on the leg ZMP measurements
%flight leg is assigned a low weight, whereas stance leg obtains a high one
%the closet the zmp is to the edge, the lower the weight is
zmp_cdf = cdf_data.zmp;
fcont_cdf = cdf_data.cont;
use_ref = 0;
if use_ref
    %ZMPs have to be expressed in the local frame !!! (CORRECT THIS BEFORE
    %USING)
    zmpL = FS_ref(1:2);
    zmpR = FS_ref(3:4);
    ftot_L = FS_ref(5);
    ftot_R = FS_ref(6);
else
   %compute the values based on the model and force measurements (LFL&LFR)
    [zmpL] = compute_local_zmp_simple(LFL.Fm,FootDataPmeas);
    [zmpR] = compute_local_zmp_simple(LFR.Fm,FootDataPmeas);
    ftot_L = sum(LFL.Fm);
    ftot_R = sum(LFR.Fm);
end

%compute weights
WL_zmp = max(0,interp2(zmp_cdf.x,zmp_cdf.y,zmp_cdf.p,zmpL(1),zmpL(2)));
WL_cont = max(0,interp1(fcont_cdf.f,fcont_cdf.p,ftot_L));

WR_zmp = max(0,interp2(zmp_cdf.x,zmp_cdf.y,zmp_cdf.p,zmpR(2),zmpR(2)));
WR_cont = max(0,interp1(fcont_cdf.f,fcont_cdf.p,ftot_R));

%kinematic weights depend on contact estimation and zmp trust region
WL = WL_zmp*WL_cont;
WR = WR_zmp*WR_cont;
Wimu = 0.3;

eps = 1e-6;
%normalise weights
W_norm1 = 1/(WR+WL+eps);
W_norm2 = 1/(Wimu+WR+WL+eps);
Wimu_vec = Wimu * [0, W_norm2, W_norm2]; %discard the first angle which is yaw (ZYX convention)
WL_vec = WL * [W_norm1, W_norm2, W_norm2];
WR_vec = WR * [W_norm1, W_norm2, W_norm2];

%fuse measurements using the computed weights
eul_fused = Wimu_vec.*rotm2eul(Rw_b_imu) + WL_vec.*rotm2eul(Rw_b_Lleg) + WR_vec.*rotm2eul(Rw_b_Rleg);
Rest_w_b = eul2rotm(eul_fused);

%% compute the position of the fb in the wcf (averaging two feet)
pest_w_b = (WL*(Hw_eeL(1:3,4)-Rest_w_b*pb_eeL)+WR*(Hw_eeR(1:3,4)-Rest_w_b*pb_eeR)) * W_norm1;

%% generate the Hwb transformation and compensate for drifts
Hest_w_b = [
    Rest_w_b,pest_w_b;
    zeros(1,3),1;
];

%compute drift transformations
HLdrift = Hw_eeL\Hest_w_b*Hb_eeL;
HRdrift = Hw_eeR\Hest_w_b*Hb_eeR;

%compensation factor (between 0 [no convg] and 1 [full comp]) - has to be
%tuned
alpha = 0.1; 
%it is correct that left and right side are inverted, as stance foot will
%not drift, however it determines how much the swing foot will
alphaL = alpha*WR;
alphaR = alpha*WL;
[HcorrL,~,~] = transformtraj(eye(4),HLdrift,[0 1],alphaL);
[HcorrR,~,~] = transformtraj(eye(4),HRdrift,[0 1],alphaR);
Hw_L_corr = Hw_eeL*HcorrL;
Hw_R_corr = Hw_eeR*HcorrR;

== matlab function bipedal_robot/Controller/Comp ==
  data: Hc2 input; twb_est input; tref output; Rwb_est input; twb_ref input; Rwb_ref input; tc1 output; tc2 output; eref output; ec1 output; ec2 output
function [tref,tc1,tc2,eref,ec1,ec2] = fcn(Hc2, twb_est,Rwb_est,twb_ref,Rwb_ref)
    tref = twb_ref;
    tc1 = twb_est;
    tc2 = Hc2(1:3,4);
    eref = rotm2eul(Rwb_ref);
    ec1 = rotm2eul(Rwb_est);
    ec2 = rotm2eul(Hc2(1:3,1:3));
